simulink model "dxdy3_sim"  (R2019a)
settings: Solver=VariableStepAuto  StartTime=0.0  StopTime=10.0  RelTol=1e-3
settings Model: Creator=hanabusa  LastModifiedBy=hanabusa

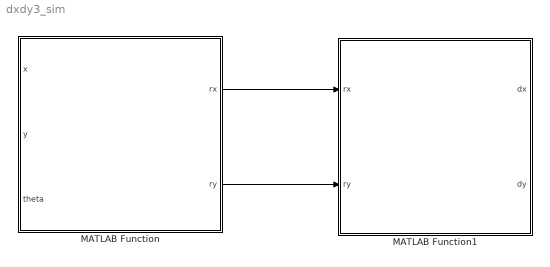
== system dxdy3_sim ==
  MATLAB Function : MATLAB Function  TreatAsAtomicUnit=on
  MATLAB Function1 : MATLAB Function  TreatAsAtomicUnit=on
  wires:
  MATLAB Function/1(rx) -> MATLAB Function1/1(rx)
  MATLAB Function/2(ry) -> MATLAB Function1/2(ry)

== matlab function dxdy3_sim/MATLAB Function1 ==
  data: dx output; rx input; dy output; ry input
function [dx,dy]=dxdy3(rx,ry)
N=5;
% desired state
dp21=[-60 0];
dp31=[-30*sqrt(3) 30];
dp32=[-30*sqrt(3) -30];
dp41=[-30*sqrt(3) -30];
dp43=[0 -60];
dp51=[-60 0];
dp54=[-30 -30*sqrt(3)];

dd=zeros(N,N); %目標の相対距離
for i=2:N    
  dd=[0 0 0 0 0;
      norm(dp21) 0 0 0 0;
      norm(dp31) norm(dp32) 0 0 0;
      norm(dp41) 0 norm(dp43) 0 0;
      norm(dp51) 0 0 norm(dp54) 0];
end
dx=zeros(1,N);    %目標位置
dy=zeros(1,N);
sgn=1; %目標の隣接順序 符号を変えれば反転する
%%
 dx(2)=rx(2,1)+dd(2,1);
 dy(2)=ry(2,1);

 for i=2:N-1 %i+1が子．その隣接する点は１とi
        % 隣接点が同じ位置
        if sqrt((rx(i+1,i)-rx(i+1,1))^2+(ry(i+1,i)-ry(i+1,1))^2)==0    
            dx(i+1)=rx(i+1,i)+dd(i+1,i);
            dy(i+1);
        end
        
        % 隣接点が近すぎる
        if 0<sqrt((rx(i+1,i)-rx(i+1,1))^2+(ry(i+1,i)-ry(i+1,1))^2)&&sqrt((rx(i+1,i)-rx(i+1,1))^2+(ry(i+1,i)-ry(i+1,1))^2)<abs(dd(i+1,1)-dd(i+1,i))
            dx(i+1)=rx(i+1,i)-dd(i+1,i)*(rx(i+1,1)-rx(i+1,i))/sqrt((rx(i+1,i)-rx(i+1,1))^2+(ry(i+1,i)-ry(i+1,1))^2);
            dy(i+1)=ry(i+1,i)-dd(i+1,i)*(ry(i+1,1)-ry(i+1,i))/sqrt((rx(i+1,i)-rx(i+1,1))^2+(ry(i+1,i)-ry(i+1,1))^2);
        end
        
        % 好位置
         if abs(dd(i+1,1)-dd(i+1,i))<=sqrt((rx(i+1,i)-rx(i+1,1))^2+(ry(i+1,i)-ry(i+1,1))^2)&&sqrt((rx(i+1,i)-rx(i+1,1))^2+(ry(i+1,i)-ry(i+1,1))^2)<=abs(dd(i+1,1)+dd(i+1,i))
             costheta=(dd(i+1,i)^2+((rx(i+1,i)-rx(i+1,1))^2+(ry(i+1,i)-ry(i+1,1))^2)-dd(i+1,1)^2)/(2*dd(i+1,i)*sqrt((rx(i+1,i)-rx(i+1,1))^2+(ry(i+1,i)-ry(i+1,1))^2));
             sintheta=sqrt(1-costheta^2);
             R=[costheta sgn*sintheta; -sgn*sintheta costheta]; %回転行列
             dx(i+1)=rx(i+1,i)+(R(1,1)*(rx(i+1,1)-rx(i+1,i))+R(1,2)*(ry(i+1,1)-ry(i+1,i)))*dd(i+1,i)/(sqrt((rx(i+1,i)-rx(i+1,1))^2+(ry(i+1,i)-ry(i+1,1))^2));
             dy(i+1)=ry(i+1,i)+(R(2,1)*(rx(i+1,1)-rx(i+1,i))+R(2,2)*(ry(i+1,1)-ry(i+1,i)))*dd(i+1,i)/(sqrt((rx(i+1,i)-rx(i+1,1))^2+(ry(i+1,i)-ry(i+1,1))^2));
         end
         
        % 隣接点が遠すぎる
         if abs(dd(i+1,1)+dd(i+1,i))<sqrt((rx(i+1,i)-rx(i+1,1))^2+(ry(i+1,i)-ry(i+1,1))^2)
             dx(i+1)=rx(i+1,i)+dd(i+1,i)*(rx(i+1,1)-rx(i+1,i))/(sqrt((rx(i+1,i)-rx(i+1,1))^2+(ry(i+1,i)-ry(i+1,1))^2));
             dy(i+1)=ry(i+1,i)+dd(i+1,i)*(ry(i+1,1)-ry(i+1,i))/(sqrt((rx(i+1,i)-rx(i+1,1))^2+(ry(i+1,i)-ry(i+1,1))^2));
         end
 end
end

== matlab function dxdy3_sim/MATLAB Function ==
  data: x input; rx output; y input; theta input; ry output
function [rx,ry]=relative_position(x,y,theta)
N=5;
rx=zeros(N,N);   %相対位置　行が基準  
ry=zeros(N,N);

 for i=1:N
     for j=1:N
       rx(i,j)=cos(theta(i))*(x(j)-x(i))+sin(theta(i))*(y(j)-y(i)); %iから見たjの相対位置
       ry(i,j)=-sin(theta(i))*(x(j)-x(i))+cos(theta(i))*(y(j)-y(i));
     end
 end
end
